simulink model "vin3"  (Simulink 7.6)
settings: Solver=ode45  StartTime=0.0  StopTime=1  RelTol=1e-3
libraries: powerlib x40
settings Model: Creator=Vinod Kumar  LastModifiedBy=huanglei
settings OptimizationCC: InitFltsAndDblsToZero=on
settings DebuggingCC: SaveWithParameterizedLinksMsg=none  MultiTaskCondExecSysMsg=none  StrictBusMsg=Warning
settings RTWCC: IncludeERTFirstTime=on

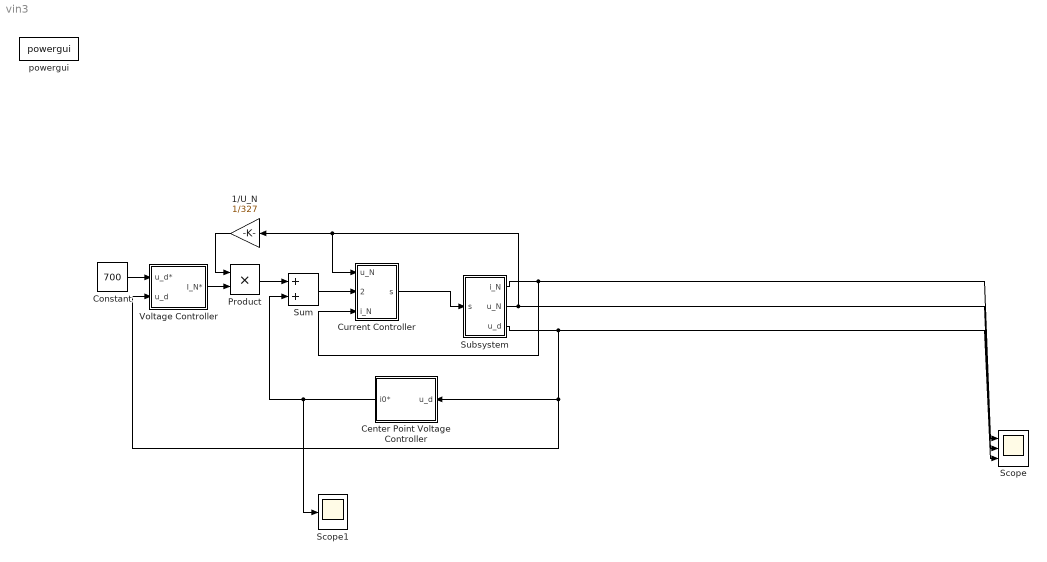
== system vin3 ==
  1/U_N : Gain  Gain=1/327
  Center Point Voltage Controller : Subsystem
  Constant : Constant  Value=700
  Current Controller : Subsystem
  Product : Product  RndMeth=Zero
  Scope : Scope  NumInputPorts=3
      settings: TimeRange=0.02  YMin=-35~-350~315  YMax=35~350~385
  Scope1 : Scope
      settings: TimeRange=1  YMin=-10000  YMax=10000  SaveName=ScopeData9
  Subsystem : Subsystem
  Sum : Sum
  Voltage Controller : Subsystem
  powergui : powerlib/powergui  SystemSampleTime=-1  SimulationMode=Continuous  SampleTime=50e-6  frequency=60  SPID=off  DisableSnubberDevices=off  DisableRonSwitches=off  DisableVfSwitches=off  SwTol=0  Interpol=off  frequencyindice=50  echomessages=off  HookPort=off  DisplayEquations=off  FunctionMessages=off  EnableUseOfTLC=off  x0status=blocks  RestoreLinks=warning  ResistiveCurrentMeasurement=off  Frange=[0:2:500]  Ylog=off  Xlog=on  ShowGrid=off  save=off  variable=ZData  ZoomFFT=on  StartTime=0.0  cycles=1  DisplayStyle=1  fundamental=60  FreqAxis=off  MaxFrequency=1000  frequencyindicesteady=1  RmsSteady=1  display=off  Ts=0  methode=off
  wires:
  Subsystem/1(i_N) -> Scope/1, Current Controller/3(i_N)
  Subsystem/2(u_N) -> Scope/2, 1/U_N/1, Current Controller/1(u_N)
  Current Controller/1(s) -> Subsystem/1(s)
  Subsystem/3(u_d) -> Voltage Controller/2(u_d), Center Point Voltage Controller/1(u_d), Scope/3
  Product/1 -> Sum/1
  Sum/1 -> Current Controller/2(i_N*)
  Constant/1 -> Voltage Controller/1(u_d*)
  1/U_N/1 -> Product/1
  Voltage Controller/1(I_N*) -> Product/2
  Center Point Voltage Controller/1(i0*) -> Sum/2, Scope1/1

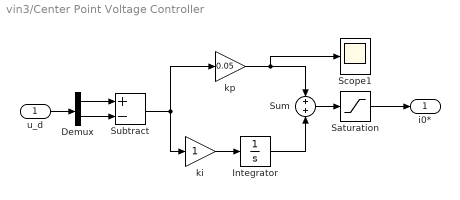
== system vin3/Center Point Voltage Controller ==
  u_d : Inport
  Demux : Demux  Outputs=2
  Integrator : Integrator  LimitOutput=on  UpperSaturationLimit=80  LowerSaturationLimit=0
  Saturation : Saturate  UpperLimit=inf  LowerLimit=-inf
  Scope1 : Scope
      settings: TimeRange=1  YMin=-10000  YMax=10000  SaveName=ScopeData11
  Subtract : Sum  Inputs=+-
  Sum : Sum  Inputs=+|+
  ki : Gain
  kp : Gain  Gain=0.05
  i0* : Outport
  wires:
  u_d/1 -> Demux/1
  Demux/1 -> Subtract/1
  Demux/2 -> Subtract/2
  Subtract/1 -> ki/1, kp/1
  ki/1 -> Integrator/1
  Integrator/1 -> Sum/2
  kp/1 -> Sum/1, Scope1/1
  Sum/1 -> Saturation/1
  Saturation/1 -> i0*/1

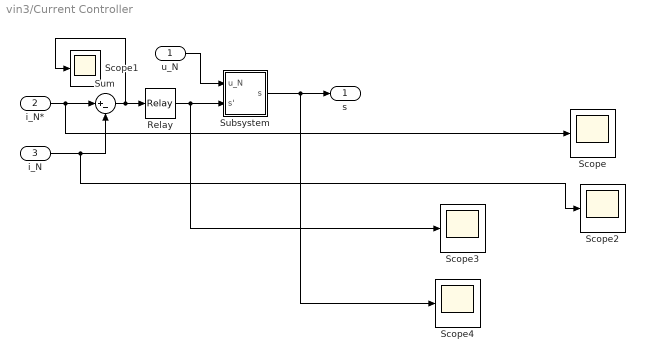
== system vin3/Current Controller ==
  u_N : Inport
  i_N* : Inport  Port=2
  i_N : Inport  Port=3
  Relay : Relay  OnSwitchValue=1.5  OffSwitchValue=-1.5
  Scope{,1..4} (5 alike) : Scope
      Scope settings: TimeRange=2e-005  YMin=-1  SaveName=ScopeData3
      Scope1 settings: TimeRange=1  YMin=-10000  YMax=10000  SaveName=ScopeData8
      Scope2 settings: TimeRange=2e-005  YMin=-1  SaveName=ScopeData12
      Scope3 settings: TimeRange=2e-005  YMin=-1  SaveName=ScopeData13
      Scope4 settings: TimeRange=2e-005  YMin=-1  SaveName=ScopeData14
  Subsystem : Subsystem
  Sum : Sum  Inputs=|+-
  s : Outport
  wires:
  Sum/1 -> Relay/1, Scope1/1
  Relay/1 -> Subsystem/2(s'), Scope3/1
  i_N*/1 -> Sum/1, Scope/1
  i_N/1 -> Sum/2, Scope2/1
  Subsystem/1(s) -> s/1, Scope4/1
  u_N/1 -> Subsystem/1(u_N)

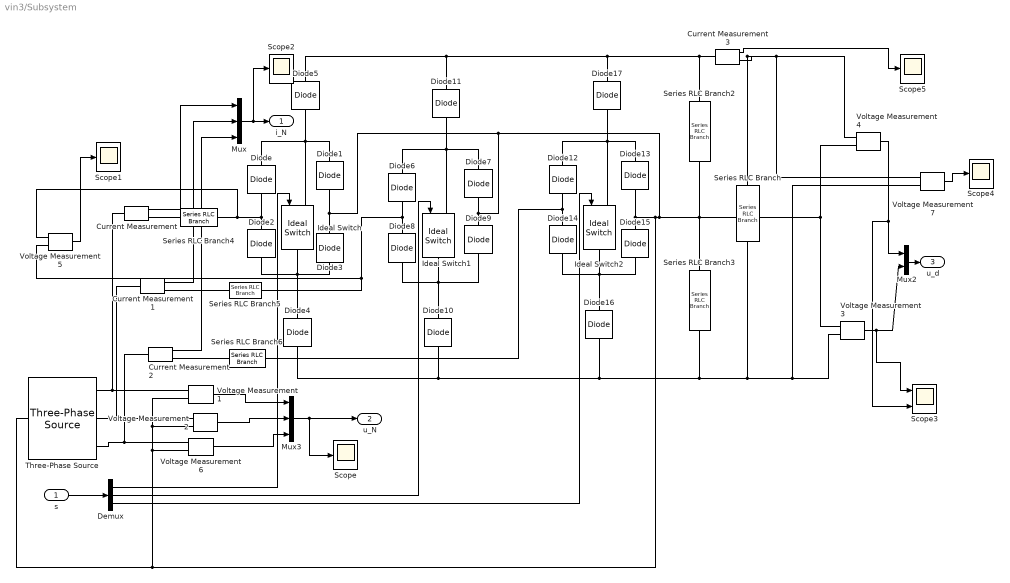
== system vin3/Subsystem ==
  s : Inport
  Current Measurement{,1..3} (4 alike) : powerlib/Measurements/Current Measurement  DialogController=POWERSYS.PowerSysDialog  SystemSampleTime=-1  PhasorSimulation=off  OutputType=Complex  PSBequivalent=0
  Demux : Demux  Outputs=3
  Diode{,1..17} (18 alike) : powerlib/Power Electronics/Diode  DialogController=POWERSYS.PowerSysDialog  SystemSampleTime=-1  Ron=0.001  Lon=0  Vf=0.8  IC=0  UseSnubber=off  Rs=500  Cs=250e-9  Measurements=off
  Ideal Switch : powerlib/Power Electronics/Ideal Switch  DialogController=POWERSYS.PowerSysDialog  SystemSampleTime=-1  Ron=0.001  Lon=0  IC=0  Rs=1e5  Cs=inf  Measurements=off
  Ideal Switch1 : powerlib/Power Electronics/Ideal Switch  DialogController=POWERSYS.PowerSysDialog  SystemSampleTime=-1  Ron=0.001  Lon=0  IC=0  Rs=1e5  Cs=inf  Measurements=off
  Ideal Switch2 : powerlib/Power Electronics/Ideal Switch  DialogController=POWERSYS.PowerSysDialog  SystemSampleTime=-1  Ron=0.001  Lon=0  IC=0  Rs=1e5  Cs=inf  Measurements=off
  Mux : Mux  Inputs=3
  Mux2 : Mux  Inputs=2
  Mux3 : Mux  Inputs=3
  Scope{,1..2,4..5} (5 alike) : Scope
      Scope settings: TimeRange=0.02  YMin=-350  YMax=350
      Scope1 settings: TimeRange=1  YMin=-10000  YMax=10000  SaveName=ScopeData2
      Scope2 settings: TimeRange=0.02  YMin=-35  YMax=35  SaveName=ScopeData4
      Scope4 settings: TimeRange=0.02  YMin=699  YMax=702.25  SaveName=ScopeData6
      Scope5 settings: TimeRange=0.02  YMin=17.47  YMax=17.5075  SaveName=ScopeData15
  Scope3 : Scope  NumInputPorts=2
      settings: TimeRange=1  YMin=374~317  YMax=383~326  SaveName=ScopeData5
  Series RLC Branch : powerlib/Elements/Series RLC Branch  DialogController=POWERSYS.PowerSysDialog  PhysicalDomain=powersysdomain  SubClassName=unknown  LeftPortType=p1  RightPortType=p1  LConnTagsString=__new0  RConnTagsString=__new0  BranchType=R  Resistance=40  Inductance=1e-3  SetiL0=off  InitialCurrent=0  Capacitance=1e-6  Setx0=off  InitialVoltage=0  Measurements=None
  Series RLC Branch2 : powerlib/Elements/Series RLC Branch  DialogController=POWERSYS.PowerSysDialog  PhysicalDomain=powersysdomain  SubClassName=unknown  LeftPortType=p1  RightPortType=p1  LConnTagsString=__new0  RConnTagsString=__new0  BranchType=C  Resistance=1  Inductance=1e-3  SetiL0=off  InitialCurrent=0  Capacitance=2000e-6  Setx0=on  InitialVoltage=300  Measurements=None
  Series RLC Branch3 : powerlib/Elements/Series RLC Branch  DialogController=POWERSYS.PowerSysDialog  PhysicalDomain=powersysdomain  SubClassName=unknown  LeftPortType=p1  RightPortType=p1  LConnTagsString=__new0  RConnTagsString=__new0  BranchType=C  Resistance=1  Inductance=1e-3  SetiL0=off  InitialCurrent=0  Capacitance=2000e-6  Setx0=on  InitialVoltage=300  Measurements=None
  Series RLC Branch4 : powerlib/Elements/Series RLC Branch  DialogController=POWERSYS.PowerSysDialog  PhysicalDomain=powersysdomain  SubClassName=unknown  LeftPortType=p1  RightPortType=p1  LConnTagsString=__new0  RConnTagsString=__new0  BranchType=L  Resistance=1  Inductance=0.3e-3  SetiL0=off  InitialCurrent=0  Capacitance=1e-6  Setx0=off  InitialVoltage=0  Measurements=None
  Series RLC Branch5 : powerlib/Elements/Series RLC Branch  DialogController=POWERSYS.PowerSysDialog  PhysicalDomain=powersysdomain  SubClassName=unknown  LeftPortType=p1  RightPortType=p1  LConnTagsString=__new0  RConnTagsString=__new0  BranchType=L  Resistance=1  Inductance=0.3e-3  SetiL0=off  InitialCurrent=0  Capacitance=1e-6  Setx0=off  InitialVoltage=0  Measurements=None
  Series RLC Branch6 : powerlib/Elements/Series RLC Branch  DialogController=POWERSYS.PowerSysDialog  PhysicalDomain=powersysdomain  SubClassName=unknown  LeftPortType=p1  RightPortType=p1  LConnTagsString=__new0  RConnTagsString=__new0  BranchType=L  Resistance=1  Inductance=0.3e-3  SetiL0=off  InitialCurrent=0  Capacitance=1e-6  Setx0=off  InitialVoltage=0  Measurements=None
  Three-Phase Source : powerlib/Electrical Sources/Three-Phase Source  DialogController=POWERSYS.PowerSysDialog  SystemSampleTime=-1  Voltage=400  PhaseAngle=0  Frequency=50  InternalConnection=Yn  SpecifyImpedance=off  Resistance=0.000001  Inductance=0  ShortCircuitLevel=100e6  BaseVoltage=25e3  XRratio=7
  Voltage Measurement{1..7} (7 alike) : powerlib/Measurements/Voltage Measurement  DialogController=POWERSYS.PowerSysDialog  SystemSampleTime=-1  PhasorSimulation=off  OutputType=Complex  PSBequivalent=0
  i_N : Outport
  u_N : Outport  Port=2
  u_d : Outport  Port=3
  wires:
  s/1 -> Demux/1
  Demux/1 -> Ideal Switch/1
  Demux/2 -> Ideal Switch1/1
  Demux/3 -> Ideal Switch2/1
  Mux/1 -> i_N/1, Scope2/1
  Voltage Measurement4/1 -> Mux2/1, Scope3/2
  Voltage Measurement3/1 -> Mux2/2, Scope3/1
  Mux2/1 -> u_d/1
  Mux3/1 -> u_N/1, Scope/1
  Voltage Measurement1/1 -> Mux3/1
  Voltage Measurement2/1 -> Mux3/2
  Current Measurement/1 -> Mux/1
  Current Measurement1/1 -> Mux/2
  Current Measurement2/1 -> Mux/3
  Voltage Measurement5/1 -> Scope1/1
  Voltage Measurement6/1 -> Mux3/3
  Voltage Measurement7/1 -> Scope4/1
  Current Measurement3/1 -> Scope5/1
  connections:
  Current Measurement/RConn1 -- Series RLC Branch4/LConn1
  Current Measurement1/RConn1 -- Series RLC Branch5/LConn1
  Current Measurement2/RConn1 -- Series RLC Branch6/LConn1
  Series RLC Branch4/RConn1 -- Diode2/RConn1 -- Diode/LConn1 -- Voltage Measurement5/LConn1
  Diode/RConn1 -- Diode1/RConn1 -- Ideal Switch/LConn1 -- Diode5/LConn1
  Series RLC Branch3/RConn1 -- Diode16/LConn1 -- Diode10/LConn1 -- Diode4/LConn1 -- Series RLC Branch/RConn1 -- Voltage Measurement3/LConn2 -- Voltage Measurement7/LConn2
  Diode10/RConn1 -- Diode9/LConn1 -- Ideal Switch1/RConn1 -- Diode8/LConn1
  Diode11/LConn1 -- Diode6/RConn1 -- Diode7/RConn1 -- Ideal Switch1/LConn1
  Series RLC Branch/LConn1 -- Voltage Measurement4/LConn1 -- Voltage Measurement7/LConn1 -- Current Measurement3/RConn1
  Diode14/RConn1 -- Diode12/LConn1 -- Series RLC Branch6/RConn1
  Diode17/LConn1 -- Diode12/RConn1 -- Diode13/RConn1 -- Ideal Switch2/LConn1
  Diode16/RConn1 -- Diode15/LConn1 -- Diode14/LConn1 -- Ideal Switch2/RConn1
  Diode2/LConn1 -- Diode3/LConn1 -- Ideal Switch/RConn1 -- Diode4/RConn1
  Diode8/RConn1 -- Diode6/LConn1 -- Series RLC Branch5/RConn1 -- Voltage Measurement5/LConn2
  Three-Phase Source/RConn1 -- Voltage Measurement1/LConn1 -- Current Measurement/LConn1
  Voltage Measurement6/LConn1 -- Three-Phase Source/RConn3 -- Current Measurement2/LConn1
  Three-Phase Source/RConn2 -- Voltage Measurement2/LConn1 -- Current Measurement1/LConn1
  Diode15/RConn1 -- Diode13/LConn1 -- Series RLC Branch2/RConn1 -- Series RLC Branch3/LConn1 -- Voltage Measurement4/LConn2 -- Voltage Measurement3/LConn1 -- Diode9/RConn1 -- Diode7/LConn1 -- Diode1/LConn1 -- Diode3/RConn1 -- Three-Phase Source/LConn1 -- Voltage Measurement1/LConn2 -- Voltage Measurement2/LConn2 -- Voltage Measurement6/LConn2
  Diode17/RConn1 -- Diode11/RConn1 -- Diode5/RConn1 -- Series RLC Branch2/LConn1 -- Current Measurement3/LConn1

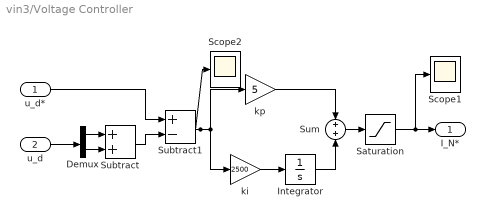
== system vin3/Voltage Controller ==
  u_d* : Inport
  u_d : Inport  Port=2
  Demux : Demux  Outputs=2
  Integrator : Integrator  LimitOutput=on  UpperSaturationLimit=80  LowerSaturationLimit=0
  Saturation : Saturate  UpperLimit=80  LowerLimit=0
  Scope1 : Scope
      settings: TimeRange=1  YMin=7.5  YMax=27.5  SaveName=ScopeData7
  Scope2 : Scope
      settings: TimeRange=1  YMin=-2.5  YMax=1  SaveName=ScopeData10
  Subtract : Sum
  Subtract1 : Sum  Inputs=+-
  Sum : Sum  Inputs=+|+
  ki : Gain  Gain=2500
  kp : Gain  Gain=5
  I_N* : Outport
  wires:
  Sum/1 -> Saturation/1
  kp/1 -> Sum/1
  Integrator/1 -> Sum/2
  ki/1 -> Integrator/1
  Demux/2 -> Subtract/2
  Demux/1 -> Subtract/1
  u_d/1 -> Demux/1
  u_d*/1 -> Subtract1/1
  Subtract/1 -> Subtract1/2
  Subtract1/1 -> ki/1, kp/1, Scope2/1
  Saturation/1 -> I_N*/1, Scope1/1

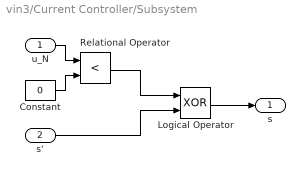
== system vin3/Current Controller/Subsystem ==
  u_N : Inport
  s' : Inport  Port=2
  Constant : Constant  Value=0
  Logical Operator : Logic  Operator=XOR  AllPortsSameDT=off  OutDataTypeStr=boolean
  Relational Operator : RelationalOperator  Operator=<  OutDataTypeStr=boolean
  s : Outport
  wires:
  Logical Operator/1 -> s/1
  u_N/1 -> Relational Operator/1
  Constant/1 -> Relational Operator/2
  Relational Operator/1 -> Logical Operator/1
  s'/1 -> Logical Operator/2
